simulink library "ammclib_bam_S32K14x"  (R2016a)
settings: Solver=VariableStepAuto  SolverMode=SingleTasking  StartTime=0.0  StopTime=10.0  RelTol=1e-3
undefined symbols (not defined in the file or in its folder): f16A1, f16A2, f16ADCMaxError, f16B0, f16B1, f16B2, f16C1, f16CC1, f16CC1sc, f16CC1sc_D, f16CC1sc_Q, f16CC2, f16CC2sc, f16CC2sc_D, f16CC2sc_Q, f16DerivGain, f16EGain, f16FiltCoef, f16HystOff, f16HystOn, f16IGain, f16IntegGain, f16IntegGainFW, f16IntegGainQ, f16Kd, f16Kq, f16Limit, f16LowerLimit, f16LowerLimit_D, f16LowerLimit_Q, f16LowerLimitFW, f16LowerLimitQ, f16ModIndex, f16OutValOff, f16OutValOn, f16PropGain, f16PropGainFW, f16PropGainQ, f16RampDown, f16RampUp, f16UGain, f16UpperLimit, f16UpperLimit_D, f16UpperLimit_Q, f16UpperLimitFW, f16UpperLimitQ, f16WIGain, f32A1, f32A2, f32ADCMaxError, f32B0, f32B1, f32B2, f32C1, f32CC1, f32CC1sc, f32CC1sc_D, f32CC1sc_Q, f32CC2, f32CC2sc ... (+114)
(part 14 of 22)

== system ammclib_bam_S32K14x/GMCLIB/F16 ==
  GMCLIB_BetaProjection3Ph_F16 : Subsystem  TreatAsAtomicUnit=on  mask(GMCLIB_BetaProjection3Ph_F16){}
      mask help: 3-phase Beta-projection transformation in 16-bit fixed-point fractional implementation. Refer to the AMMCLIB User's Guide for further details.
      mask init: same as ammclib_bam_S32K14x/GDFLIB/F16/GDFLIB_FilterFIR_F16
      settings: RTWSystemCode=Inline
      mask Help: web([fileparts(which('ammclib_bam_S32K14x.slx')) '/../doc/S32K14XMCLUG.pdf'], '-browser')
      mask Display: pos = get_param(gcb, 'Position');width = pos(3) - pos(1); height = pos(4) - pos(2);tX=width/2;tY=height - 8;color('black');text(tX,tY, 'GMCLIB_BetaProjection3Ph_F16', 'horizontalAlignment', 'center');
  GMCLIB_BetaProjection_F16 : Subsystem  TreatAsAtomicUnit=on  mask(GMCLIB_BetaProjection_F16){}
      mask help: Beta Projection transformation 3ph -> 2ph in 16-bit fixed-point fractional implementation. Refer to the AMMCLIB User's Guide for further details.
      mask init: same as ammclib_bam_S32K14x/GDFLIB/F16/GDFLIB_FilterFIR_F16
      settings: RTWSystemCode=Inline
      mask Help: web([fileparts(which('ammclib_bam_S32K14x.slx')) '/../doc/S32K14XMCLUG.pdf'], '-browser')
      mask Display: pos = get_param(gcb, 'Position');width = pos(3) - pos(1); height = pos(4) - pos(2);tX=width/2;tY=height - 8;color('black');text(tX,tY, 'GMCLIB_BetaProjection_F16', 'horizontalAlignment', 'center');
  GMCLIB_ClarkInv_F16 : Subsystem  TreatAsAtomicUnit=on  mask(GMCLIB_ClarkInv_F16){}
      mask help: Inverse Clarke transformation 2ph -> 3ph in 16-bit fixed-point fractional implementation. Refer to the AMMCLIB User's Guide for further details.
      mask init: same as ammclib_bam_S32K14x/GDFLIB/F16/GDFLIB_FilterFIR_F16
      settings: RTWSystemCode=Inline
      mask Help: web([fileparts(which('ammclib_bam_S32K14x.slx')) '/../doc/S32K14XMCLUG.pdf'], '-browser')
      mask Display: pos = get_param(gcb, 'Position');width = pos(3) - pos(1); height = pos(4) - pos(2);tX=width/2;tY=height - 8;color('black');text(tX,tY, 'GMCLIB_ClarkInv_F16', 'horizontalAlignment', 'center');
  GMCLIB_Clark_F16 : Subsystem  TreatAsAtomicUnit=on  mask(GMCLIB_Clark_F16){}
      mask help: Clarke transformation 3ph -> 2ph in 16-bit fixed-point fractional implementation. Refer to the AMMCLIB User's Guide for further details.
      mask init: same as ammclib_bam_S32K14x/GDFLIB/F16/GDFLIB_FilterFIR_F16
      settings: RTWSystemCode=Inline
      mask Help: web([fileparts(which('ammclib_bam_S32K14x.slx')) '/../doc/S32K14XMCLUG.pdf'], '-browser')
      mask Display: pos = get_param(gcb, 'Position');width = pos(3) - pos(1); height = pos(4) - pos(2);tX=width/2;tY=height - 8;color('black');text(tX,tY, 'GMCLIB_Clark_F16', 'horizontalAlignment', 'center');
  GMCLIB_DecouplingPMSM_F16 : Subsystem  TreatAsAtomicUnit=on  mask(GMCLIB_DecouplingPMSM_F16){showStates=Hide (faster execution), f16Kd=0, s16KdShift=0, f16Kq=0, s16KqShift=0}
      mask prompts: showStates "Show internal states"; f16Kd "f16Kd (Coefficient k_d)"; s16KdShift "s16KdShift (Scaling coefficient k_d_shift)"; f16Kq "f16Kq (Coefficient k_q)"; s16KqShift "s16KqShift (Scaling coefficient k_q_shift)"
      mask help: Decoupling of d and q axis of PMSM model in 16-bit fixed-point fractional implementation. Refer to the AMMCLIB User's Guide for further details.
      mask init:
      | if ~evalin('base','exist(''tS8'',''var'')')
      |   if (2 ~= exist('SWLIBS_Typedefs.mat','file'))
      |       error('File SWLIBS_Typedefs.mat is not on the Matlab path. Please add the AMMCLIB "bam" folder in the Matlab Search Path.');
      |   else
      |       evalin('base', 'load(''SWLIBS_Typedefs.mat'')');
      |   end
      | end
      | if showStates == 1
      |     % hidden state variables
      |     if strcmp(get_param([gcb '/f16Kd'], 'BlockType'), 'Inport')
      |         posblk = get_param(gcb, 'Position');
      | 
      |         pos = get_param(    [gcb, '/f16Kd'], 'Position');
      |         orient = get_param( [gcb, '/f16Kd'], 'Orientation');
      |         delete_block(       [gcb, '/f16Kd']);
      |         add_block('built-in/Ground', [gcb, '/f16Kd'], 'Position', pos, 'Orientation', orient);
      | 
      |         pos = get_param(    [gcb, '/s16KdShift'], 'Position');
      |         orient = get_param( [gcb, '/s16KdShift'], 'Orientation');
      |         delete_block(       [gcb, '/s16KdShift']);
      |         add_block('built-in/Ground', [gcb, '/s16KdShift'], 'Position', pos, 'Orientation', orient);
      | 
      |         pos = get_param(    [gcb, '/f16Kq'], 'Position');
      |         orient = get_param( [gcb, '/f16Kq'], 'Orientation');
      |         delete_block(       [gcb, '/f16Kq']);
      |         add_block('built-in/Ground', [gcb, '/f16Kq'], 'Position', pos, 'Orientation', orient);
      | 
      |         pos = get_param(    [gcb, '/s16KqShift'], 'Position');
      |         orient = get_param( [gcb, '/s16KqShift'], 'Orientation');
      |         delete_block(       [gcb, '/s16KqShift']);
      |         add_block('built-in/Ground', [gcb, '/s16KqShift'], 'Position', pos, 'Orientation', orient);
      | 
      | 
      | 
      |         set_param([gcb '/pUdq'], 'Port', '1');
      |         set_param([gcb '/pIdq'], 'Port', '2');
      |         set_param([gcb '/f16AngularVel'], 'Port', '3');
      | 
      |         set_param([gcb '/pUdqDec'], 'Port', '1');
      | 
      |         set_param(gcb,'MaskEnables',{'on','on','on','on','on'});
      | 
      |         if (posblk(4) - posblk(2)) > 100
      |           height = 100;
      |           set_param(gcb,'Position',[posblk(1), posblk(2), posblk(3), posblk(2)+height])
      |         end
      |     end
      | else
      |     % shown state variables
      |     if strcmp(get_param([gcb '/f16Kd'], 'BlockType'), 'Ground')
      |         posblk = get_param(gcb, 'Position');
      | 
      |         pos = get_param(    [gcb, '/f16Kd'], 'Position');
      |         orient = get_param( [gcb, '/f16Kd'], 'Orientation');
      |         delete_block(       [gcb, '/f16Kd']);
      |         add_block('built-in/Inport', [gcb, '/f16Kd'], 'Position', pos, 'Orientation', orient, 'OutDataTypeStr', 'int16');
      | 
      |         pos = get_param(    [gcb, '/s16KdShift'], 'Position');
      |         orient = get_param( [gcb, '/s16KdShift'], 'Orientation');
      |         delete_block(       [gcb, '/s16KdShift']);
      |         add_block('built-in/Inport', [gcb, '/s16KdShift'], 'Position', pos, 'Orientation', orient, 'OutDataTypeStr', 'int16');
      | 
      |         pos = get_param(    [gcb, '/f16Kq'], 'Position');
      |         orient = get_param( [gcb, '/f16Kq'], 'Orientation');
      |         delete_block(       [gcb, '/f16Kq']);
      |         add_block('built-in/Inport', [gcb, '/f16Kq'], 'Position', pos, 'Orientation', orient, 'OutDataTypeStr', 'int16');
      | 
      |         pos = get_param(    [gcb, '/s16KqShift'], 'Position');
      |         orient = get_param( [gcb, '/s16KqShift'], 'Orientation');
      |         delete_block(       [gcb, '/s16KqShift']);
      |         add_block('built-in/Inport', [gcb, '/s16KqShift'], 'Position', pos, 'Orientation', orient, 'OutDataTypeStr', 'int16');
      | 
      | 
      | 
      |         set_param([gcb '/pUdq'], 'Port', '1');
      |         set_param([gcb '/pIdq'], 'Port', '2');
      |         set_param([gcb '/f16AngularVel'], 'Port', '3');
      |         set_param([gcb '/f16Kd'], 'Port', '4');
      |         set_param([gcb '/s16KdShift'], 'Port', '5');
      |         set_param([gcb '/f16Kq'], 'Port', '6');
      |         set_param([gcb '/s16KqShift'], 'Port', '7');
      | 
      |         set_param([gcb '/pUdqDec'], 'Port', '1');
      | 
      |         set_param(gcb,'MaskEnables',{'on','off','off','off','off'});
      | 
      |         if (posblk(4) - posblk(2)) < 200
      |           height = 200;
      |           set_param(gcb,'Position',[posblk(1), posblk(2), posblk(3), posblk(2)+height])
      |         end
      |     end
      | end
      settings: RTWSystemCode=Inline
      mask Help: web([fileparts(which('ammclib_bam_S32K14x.slx')) '/../doc/S32K14XMCLUG.pdf'], '-browser')
      mask TypeOptions showStates: Hide (faster execution) | Show (allows debugging; connect feedback loops manually)
      mask Callback showStates:
      | maskStr = get_param(gcb,'showStates');
      | if strcmp(maskStr,'Hide (faster execution)'),
      |     set_param(gcb,'MaskEnables',{'on','on','on','on','on'});
      | else
      |     set_param(gcb,'MaskEnables',{'on','off','off','off','off'});
      | end
      mask Display:
      | color('black');
      | pos = get_param(gcb, 'Position');
      | width = pos(3) - pos(1);
      | height = pos(4) - pos(2);
      | tX=width/2;
      | tY=height - 8;
      | color('black');
      | text(tX,tY, 'GMCLIB_DecouplingPMSM_F16', 'horizontalAlignment', 'center');
      | if showStates == 2
      |   color('red');
      |   text(tX,tY - 20, ['debugging mode' char(13) char(10) '(limited performance)'], 'horizontalAlignment', 'center');
      | end
  GMCLIB_ElimDcBusRip_F16 : Subsystem  TreatAsAtomicUnit=on  mask(GMCLIB_ElimDcBusRip_F16){showStates=Hide (faster execution), f16ModIndex=0}
      mask prompts: showStates "Show internal states"; f16ModIndex "f16ModIndex (Inverse Modulation Index)"
      mask help: DC Bus voltage ripple elimination function in 16-bit fixed-point fractional implementation. Refer to the AMMCLIB User's Guide for further details.
      mask init:
      | if ~evalin('base','exist(''tS8'',''var'')')
      |   if (2 ~= exist('SWLIBS_Typedefs.mat','file'))
      |       error('File SWLIBS_Typedefs.mat is not on the Matlab path. Please add the AMMCLIB "bam" folder in the Matlab Search Path.');
      |   else
      |       evalin('base', 'load(''SWLIBS_Typedefs.mat'')');
      |   end
      | end
      | if showStates == 1
      |     % hidden state variables
      |     if strcmp(get_param([gcb '/f16ModIndex'], 'BlockType'), 'Inport')
      |         posblk = get_param(gcb, 'Position');
      | 
      |         pos = get_param(    [gcb, '/f16ModIndex'], 'Position');
      |         orient = get_param( [gcb, '/f16ModIndex'], 'Orientation');
      |         delete_block(       [gcb, '/f16ModIndex']);
      |         add_block('built-in/Ground', [gcb, '/f16ModIndex'], 'Position', pos, 'Orientation', orient);
      | 
      | 
      | 
      |         set_param([gcb '/pIn'], 'Port', '1');
      |         set_param([gcb '/f16ArgDcBusMsr'], 'Port', '2');
      | 
      |         set_param([gcb '/pOut'], 'Port', '1');
      | 
      |         set_param(gcb,'MaskEnables',{'on','on'});
      | 
      |         if (posblk(4) - posblk(2)) > 75
      |           height = 75;
      |           set_param(gcb,'Position',[posblk(1), posblk(2), posblk(3), posblk(2)+height])
      |         end
      |     end
      | else
      |     % shown state variables
      |     if strcmp(get_param([gcb '/f16ModIndex'], 'BlockType'), 'Ground')
      |         posblk = get_param(gcb, 'Position');
      | 
      |         pos = get_param(    [gcb, '/f16ModIndex'], 'Position');
      |         orient = get_param( [gcb, '/f16ModIndex'], 'Orientation');
      |         delete_block(       [gcb, '/f16ModIndex']);
      |         add_block('built-in/Inport', [gcb, '/f16ModIndex'], 'Position', pos, 'Orientation', orient, 'OutDataTypeStr', 'int16');
      | 
      | 
      | 
      |         set_param([gcb '/pIn'], 'Port', '1');
      |         set_param([gcb '/f16ArgDcBusMsr'], 'Port', '2');
      |         set_param([gcb '/f16ModIndex'], 'Port', '3');
      | 
      |         set_param([gcb '/pOut'], 'Port', '1');
      | 
      |         set_param(gcb,'MaskEnables',{'on','off'});
      | 
      |         if (posblk(4) - posblk(2)) < 100
      |           height = 100;
      |           set_param(gcb,'Position',[posblk(1), posblk(2), posblk(3), posblk(2)+height])
      |         end
      |     end
      | end
      settings: RTWSystemCode=Inline
      mask Help: web([fileparts(which('ammclib_bam_S32K14x.slx')) '/../doc/S32K14XMCLUG.pdf'], '-browser')
      mask TypeOptions showStates: Hide (faster execution) | Show (allows debugging; connect feedback loops manually)
      mask Callback showStates:
      | maskStr = get_param(gcb,'showStates');
      | if strcmp(maskStr,'Hide (faster execution)'),
      |     set_param(gcb,'MaskEnables',{'on','on'});
      | else
      |     set_param(gcb,'MaskEnables',{'on','off'});
      | end
      mask Display:
      | color('black');
      | pos = get_param(gcb, 'Position');
      | width = pos(3) - pos(1);
      | height = pos(4) - pos(2);
      | tX=width/2;
      | tY=height - 8;
      | color('black');
      | text(tX,tY, 'GMCLIB_ElimDcBusRip_F16', 'horizontalAlignment', 'center');
      | if showStates == 2
      |   color('red');
      |   text(tX,tY - 20, ['debugging mode' char(13) char(10) '(limited performance)'], 'horizontalAlignment', 'center');
      | end
  GMCLIB_ParkInv_F16 : Subsystem  TreatAsAtomicUnit=on  mask(GMCLIB_ParkInv_F16){}
      mask help: Inverse Park transformation 2ph rotational -> 2ph stationary in 16-bit fixed-point fractional implementation. Refer to the AMMCLIB User's Guide for further details.
      mask init: same as ammclib_bam_S32K14x/GDFLIB/F16/GDFLIB_FilterFIR_F16
      settings: RTWSystemCode=Inline
      mask Help: web([fileparts(which('ammclib_bam_S32K14x.slx')) '/../doc/S32K14XMCLUG.pdf'], '-browser')
      mask Display: pos = get_param(gcb, 'Position');width = pos(3) - pos(1); height = pos(4) - pos(2);tX=width/2;tY=height - 8;color('black');text(tX,tY, 'GMCLIB_ParkInv_F16', 'horizontalAlignment', 'center');
  GMCLIB_Park_F16 : Subsystem  TreatAsAtomicUnit=on  mask(GMCLIB_Park_F16){}
      mask help: Park transformation 2ph stationary -> 2ph rotational in 16-bit fixed-point fractional implementation. Refer to the AMMCLIB User's Guide for further details.
      mask init: same as ammclib_bam_S32K14x/GDFLIB/F16/GDFLIB_FilterFIR_F16
      settings: RTWSystemCode=Inline
      mask Help: web([fileparts(which('ammclib_bam_S32K14x.slx')) '/../doc/S32K14XMCLUG.pdf'], '-browser')
      mask Display: pos = get_param(gcb, 'Position');width = pos(3) - pos(1); height = pos(4) - pos(2);tX=width/2;tY=height - 8;color('black');text(tX,tY, 'GMCLIB_Park_F16', 'horizontalAlignment', 'center');
  GMCLIB_PwmIct_F16 : Subsystem  TreatAsAtomicUnit=on  mask(GMCLIB_PwmIct_F16){}
      mask help: General Sinusoidal PWM in 16-bit fixed-point fractional implementation. Refer to the AMMCLIB User's Guide for further details.
      mask init: same as ammclib_bam_S32K14x/GDFLIB/F16/GDFLIB_FilterFIR_F16
      settings: RTWSystemCode=Inline
      mask Help: web([fileparts(which('ammclib_bam_S32K14x.slx')) '/../doc/S32K14XMCLUG.pdf'], '-browser')
      mask Display: pos = get_param(gcb, 'Position');width = pos(3) - pos(1); height = pos(4) - pos(2);tX=width/2;tY=height - 8;color('black');text(tX,tY, 'GMCLIB_PwmIct_F16', 'horizontalAlignment', 'center');
  GMCLIB_SvmSci_F16 : Subsystem  TreatAsAtomicUnit=on  mask(GMCLIB_SvmSci_F16){}
      mask help: General Sinusoidal Modulation with Injection of Third Harmonic in 16-bit fixed-point fractional implementation. Refer to the AMMCLIB User's Guide for further details.
      mask init: same as ammclib_bam_S32K14x/GDFLIB/F16/GDFLIB_FilterFIR_F16
      settings: RTWSystemCode=Inline
      mask Help: web([fileparts(which('ammclib_bam_S32K14x.slx')) '/../doc/S32K14XMCLUG.pdf'], '-browser')
      mask Display: pos = get_param(gcb, 'Position');width = pos(3) - pos(1); height = pos(4) - pos(2);tX=width/2;tY=height - 8;color('black');text(tX,tY, 'GMCLIB_SvmSci_F16', 'horizontalAlignment', 'center');
  GMCLIB_SvmStd_F16 : Subsystem  TreatAsAtomicUnit=on  mask(GMCLIB_SvmStd_F16){}
      mask help: Standard Space Vector Modulation in 16-bit fixed-point fractional implementation. Refer to the AMMCLIB User's Guide for further details.
      mask init: same as ammclib_bam_S32K14x/GDFLIB/F16/GDFLIB_FilterFIR_F16
      settings: RTWSystemCode=Inline
      mask Help: web([fileparts(which('ammclib_bam_S32K14x.slx')) '/../doc/S32K14XMCLUG.pdf'], '-browser')
      mask Display: pos = get_param(gcb, 'Position');width = pos(3) - pos(1); height = pos(4) - pos(2);tX=width/2;tY=height - 8;color('black');text(tX,tY, 'GMCLIB_SvmStd_F16', 'horizontalAlignment', 'center');
  GMCLIB_SvmU0n_F16 : Subsystem  TreatAsAtomicUnit=on  mask(GMCLIB_SvmU0n_F16){}
      mask help: Special Space Vector Modulation with O_000 Nulls in 16-bit fixed-point fractional implementation. Refer to the AMMCLIB User's Guide for further details.
      mask init: same as ammclib_bam_S32K14x/GDFLIB/F16/GDFLIB_FilterFIR_F16
      settings: RTWSystemCode=Inline
      mask Help: web([fileparts(which('ammclib_bam_S32K14x.slx')) '/../doc/S32K14XMCLUG.pdf'], '-browser')
      mask Display: pos = get_param(gcb, 'Position');width = pos(3) - pos(1); height = pos(4) - pos(2);tX=width/2;tY=height - 8;color('black');text(tX,tY, 'GMCLIB_SvmU0n_F16', 'horizontalAlignment', 'center');
  GMCLIB_SvmU7n_F16 : Subsystem  TreatAsAtomicUnit=on  mask(GMCLIB_SvmU7n_F16){}
      mask help: Special Space Vector Modulation with O_111 Ones in 16-bit fixed-point fractional implementation. Refer to the AMMCLIB User's Guide for further details.
      mask init: same as ammclib_bam_S32K14x/GDFLIB/F16/GDFLIB_FilterFIR_F16
      settings: RTWSystemCode=Inline
      mask Help: web([fileparts(which('ammclib_bam_S32K14x.slx')) '/../doc/S32K14XMCLUG.pdf'], '-browser')
      mask Display: pos = get_param(gcb, 'Position');width = pos(3) - pos(1); height = pos(4) - pos(2);tX=width/2;tY=height - 8;color('black');text(tX,tY, 'GMCLIB_SvmU7n_F16', 'horizontalAlignment', 'center');
  GMCLIB_VRot_F16 : Subsystem  TreatAsAtomicUnit=on  mask(GMCLIB_VRot_F16){}
      mask help: Vector rotation in 16-bit fixed-point fractional implementation.
      mask init: same as ammclib_bam_S32K14x/GDFLIB/F16/GDFLIB_FilterFIR_F16
      settings: RTWSystemCode=Inline
      mask Help: web([fileparts(which('ammclib_bam_S32K14x.slx')) '/../doc/S32K14XMCLUG.pdf'], '-browser')
      mask Display: pos = get_param(gcb, 'Position');width = pos(3) - pos(1); height = pos(4) - pos(2);tX=width/2;tY=height - 8;color('black');text(tX,tY, 'GMCLIB_VRot_F16', 'horizontalAlignment', 'center');
  GMCLIB_VUnit_F16 : Subsystem  TreatAsAtomicUnit=on  mask(GMCLIB_VUnit_F16){}
      mask help: Vector normalization in 16-bit fixed-point fractional implementation.
      mask init: same as ammclib_bam_S32K14x/GDFLIB/F16/GDFLIB_FilterFIR_F16
      settings: RTWSystemCode=Inline
      mask Help: web([fileparts(which('ammclib_bam_S32K14x.slx')) '/../doc/S32K14XMCLUG.pdf'], '-browser')
      mask Display: pos = get_param(gcb, 'Position');width = pos(3) - pos(1); height = pos(4) - pos(2);tX=width/2;tY=height - 8;color('black');text(tX,tY, 'GMCLIB_VUnit_F16', 'horizontalAlignment', 'center');
  GMCLIB_Vpol2xy_F16 : Subsystem  TreatAsAtomicUnit=on  mask(GMCLIB_Vpol2xy_F16){}
      mask help: Transformation of polar coordinate system to Cartesian in 16-bit fixed-point fractional implementation.
      mask init: same as ammclib_bam_S32K14x/GDFLIB/F16/GDFLIB_FilterFIR_F16
      settings: RTWSystemCode=Inline
      mask Help: web([fileparts(which('ammclib_bam_S32K14x.slx')) '/../doc/S32K14XMCLUG.pdf'], '-browser')
      mask Display: pos = get_param(gcb, 'Position');width = pos(3) - pos(1); height = pos(4) - pos(2);tX=width/2;tY=height - 8;color('black');text(tX,tY, 'GMCLIB_Vpol2xy_F16', 'horizontalAlignment', 'center');
  GMCLIB_Vxy2pol_F16 : Subsystem  TreatAsAtomicUnit=on  mask(GMCLIB_Vxy2pol_F16){}
      mask help: Transformation of Cartesian coordinate system to polar in 16-bit fixed-point fractional implementation.
      mask init: same as ammclib_bam_S32K14x/GDFLIB/F16/GDFLIB_FilterFIR_F16
      settings: RTWSystemCode=Inline
      mask Help: web([fileparts(which('ammclib_bam_S32K14x.slx')) '/../doc/S32K14XMCLUG.pdf'], '-browser')
      mask Display: pos = get_param(gcb, 'Position');width = pos(3) - pos(1); height = pos(4) - pos(2);tX=width/2;tY=height - 8;color('black');text(tX,tY, 'GMCLIB_Vxy2pol_F16', 'horizontalAlignment', 'center');

== system ammclib_bam_S32K14x/GMCLIB/F32 ==
  GMCLIB_BetaProjection3Ph_F32 : Subsystem  TreatAsAtomicUnit=on  mask(GMCLIB_BetaProjection3Ph_F32){}
      mask help: 3-phase Beta-projection transformation in 32-bit fixed-point fractional implementation. Refer to the AMMCLIB User's Guide for further details.
      mask init: same as ammclib_bam_S32K14x/GDFLIB/F16/GDFLIB_FilterFIR_F16
      settings: RTWSystemCode=Inline
      mask Help: web([fileparts(which('ammclib_bam_S32K14x.slx')) '/../doc/S32K14XMCLUG.pdf'], '-browser')
      mask Display: pos = get_param(gcb, 'Position');width = pos(3) - pos(1); height = pos(4) - pos(2);tX=width/2;tY=height - 8;color('black');text(tX,tY, 'GMCLIB_BetaProjection3Ph_F32', 'horizontalAlignment', 'center');
  GMCLIB_BetaProjection_F32 : Subsystem  TreatAsAtomicUnit=on  mask(GMCLIB_BetaProjection_F32){}
      mask help: Beta Projection transformation 3ph -> 2ph in 32-bit fixed-point fractional implementation. Refer to the AMMCLIB User's Guide for further details.
      mask init: same as ammclib_bam_S32K14x/GDFLIB/F16/GDFLIB_FilterFIR_F16
      settings: RTWSystemCode=Inline
      mask Help: web([fileparts(which('ammclib_bam_S32K14x.slx')) '/../doc/S32K14XMCLUG.pdf'], '-browser')
      mask Display: pos = get_param(gcb, 'Position');width = pos(3) - pos(1); height = pos(4) - pos(2);tX=width/2;tY=height - 8;color('black');text(tX,tY, 'GMCLIB_BetaProjection_F32', 'horizontalAlignment', 'center');
  GMCLIB_ClarkInv_F32 : Subsystem  TreatAsAtomicUnit=on  mask(GMCLIB_ClarkInv_F32){}
      mask help: Inverse Clarke transformation 2ph -> 3ph in 32-bit fixed-point fractional implementation. Refer to the AMMCLIB User's Guide for further details.
      mask init: same as ammclib_bam_S32K14x/GDFLIB/F16/GDFLIB_FilterFIR_F16
      settings: RTWSystemCode=Inline
      mask Help: web([fileparts(which('ammclib_bam_S32K14x.slx')) '/../doc/S32K14XMCLUG.pdf'], '-browser')
      mask Display: pos = get_param(gcb, 'Position');width = pos(3) - pos(1); height = pos(4) - pos(2);tX=width/2;tY=height - 8;color('black');text(tX,tY, 'GMCLIB_ClarkInv_F32', 'horizontalAlignment', 'center');
  GMCLIB_Clark_F32 : Subsystem  TreatAsAtomicUnit=on  mask(GMCLIB_Clark_F32){}
      mask help: Clarke transformation 3ph -> 2ph in 32-bit fixed-point fractional implementation. Refer to the AMMCLIB User's Guide for further details.
      mask init: same as ammclib_bam_S32K14x/GDFLIB/F16/GDFLIB_FilterFIR_F16
      settings: RTWSystemCode=Inline
      mask Help: web([fileparts(which('ammclib_bam_S32K14x.slx')) '/../doc/S32K14XMCLUG.pdf'], '-browser')
      mask Display: pos = get_param(gcb, 'Position');width = pos(3) - pos(1); height = pos(4) - pos(2);tX=width/2;tY=height - 8;color('black');text(tX,tY, 'GMCLIB_Clark_F32', 'horizontalAlignment', 'center');
  GMCLIB_DecouplingPMSM_F32 : Subsystem  TreatAsAtomicUnit=on  mask(GMCLIB_DecouplingPMSM_F32){showStates=Hide (faster execution), f32Kd=0, s16KdShift=0, f32Kq=0, s16KqShift=0}
      mask prompts: showStates "Show internal states"; f32Kd "f32Kd (Coefficient k_d)"; s16KdShift "s16KdShift (Scaling coefficient k_d_shift)"; f32Kq "f32Kq (Coefficient k_q)"; s16KqShift "s16KqShift (Scaling coefficient k_q_shift)"
      mask help: Decoupling of d and q axis of PMSM model in 32-bit fixed-point fractional implementation. Refer to the AMMCLIB User's Guide for further details.
      mask init:
      | if ~evalin('base','exist(''tS8'',''var'')')
      |   if (2 ~= exist('SWLIBS_Typedefs.mat','file'))
      |       error('File SWLIBS_Typedefs.mat is not on the Matlab path. Please add the AMMCLIB "bam" folder in the Matlab Search Path.');
      |   else
      |       evalin('base', 'load(''SWLIBS_Typedefs.mat'')');
      |   end
      | end
      | if showStates == 1
      |     % hidden state variables
      |     if strcmp(get_param([gcb '/f32Kd'], 'BlockType'), 'Inport')
      |         posblk = get_param(gcb, 'Position');
      | 
      |         pos = get_param(    [gcb, '/f32Kd'], 'Position');
      |         orient = get_param( [gcb, '/f32Kd'], 'Orientation');
      |         delete_block(       [gcb, '/f32Kd']);
      |         add_block('built-in/Ground', [gcb, '/f32Kd'], 'Position', pos, 'Orientation', orient);
      | 
      |         pos = get_param(    [gcb, '/s16KdShift'], 'Position');
      |         orient = get_param( [gcb, '/s16KdShift'], 'Orientation');
      |         delete_block(       [gcb, '/s16KdShift']);
      |         add_block('built-in/Ground', [gcb, '/s16KdShift'], 'Position', pos, 'Orientation', orient);
      | 
      |         pos = get_param(    [gcb, '/f32Kq'], 'Position');
      |         orient = get_param( [gcb, '/f32Kq'], 'Orientation');
      |         delete_block(       [gcb, '/f32Kq']);
      |         add_block('built-in/Ground', [gcb, '/f32Kq'], 'Position', pos, 'Orientation', orient);
      | 
      |         pos = get_param(    [gcb, '/s16KqShift'], 'Position');
      |         orient = get_param( [gcb, '/s16KqShift'], 'Orientation');
      |         delete_block(       [gcb, '/s16KqShift']);
      |         add_block('built-in/Ground', [gcb, '/s16KqShift'], 'Position', pos, 'Orientation', orient);
      | 
      | 
      | 
      |         set_param([gcb '/pUdq'], 'Port', '1');
      |         set_param([gcb '/pIdq'], 'Port', '2');
      |         set_param([gcb '/f32AngularVel'], 'Port', '3');
      | 
      |         set_param([gcb '/pUdqDec'], 'Port', '1');
      | 
      |         set_param(gcb,'MaskEnables',{'on','on','on','on','on'});
      | 
      |         if (posblk(4) - posblk(2)) > 100
      |           height = 100;
      |           set_param(gcb,'Position',[posblk(1), posblk(2), posblk(3), posblk(2)+height])
      |         end
      |     end
      | else
      |     % shown state variables
      |     if strcmp(get_param([gcb '/f32Kd'], 'BlockType'), 'Ground')
      |         posblk = get_param(gcb, 'Position');
      | 
      |         pos = get_param(    [gcb, '/f32Kd'], 'Position');
      |         orient = get_param( [gcb, '/f32Kd'], 'Orientation');
      |         delete_block(       [gcb, '/f32Kd']);
      |         add_block('built-in/Inport', [gcb, '/f32Kd'], 'Position', pos, 'Orientation', orient, 'OutDataTypeStr', 'int32');
      | 
      |         pos = get_param(    [gcb, '/s16KdShift'], 'Position');
      |         orient = get_param( [gcb, '/s16KdShift'], 'Orientation');
      |         delete_block(       [gcb, '/s16KdShift']);
      |         add_block('built-in/Inport', [gcb, '/s16KdShift'], 'Position', pos, 'Orientation', orient, 'OutDataTypeStr', 'int16');
      | 
      |         pos = get_param(    [gcb, '/f32Kq'], 'Position');
      |         orient = get_param( [gcb, '/f32Kq'], 'Orientation');
      |         delete_block(       [gcb, '/f32Kq']);
      |         add_block('built-in/Inport', [gcb, '/f32Kq'], 'Position', pos, 'Orientation', orient, 'OutDataTypeStr', 'int32');
      | 
      |         pos = get_param(    [gcb, '/s16KqShift'], 'Position');
      |         orient = get_param( [gcb, '/s16KqShift'], 'Orientation');
      |         delete_block(       [gcb, '/s16KqShift']);
      |         add_block('built-in/Inport', [gcb, '/s16KqShift'], 'Position', pos, 'Orientation', orient, 'OutDataTypeStr', 'int16');
      | 
      | 
      | 
      |         set_param([gcb '/pUdq'], 'Port', '1');
      |         set_param([gcb '/pIdq'], 'Port', '2');
      |         set_param([gcb '/f32AngularVel'], 'Port', '3');
      |         set_param([gcb '/f32Kd'], 'Port', '4');
      |         set_param([gcb '/s16KdShift'], 'Port', '5');
      |         set_param([gcb '/f32Kq'], 'Port', '6');
      |         set_param([gcb '/s16KqShift'], 'Port', '7');
      | 
      |         set_param([gcb '/pUdqDec'], 'Port', '1');
      | 
      |         set_param(gcb,'MaskEnables',{'on','off','off','off','off'});
      | 
      |         if (posblk(4) - posblk(2)) < 200
      |           height = 200;
      |           set_param(gcb,'Position',[posblk(1), posblk(2), posblk(3), posblk(2)+height])
      |         end
      |     end
      | end
      settings: RTWSystemCode=Inline
      mask Help: web([fileparts(which('ammclib_bam_S32K14x.slx')) '/../doc/S32K14XMCLUG.pdf'], '-browser')
      mask TypeOptions showStates: Hide (faster execution) | Show (allows debugging; connect feedback loops manually)
      mask Callback showStates:
      | maskStr = get_param(gcb,'showStates');
      | if strcmp(maskStr,'Hide (faster execution)'),
      |     set_param(gcb,'MaskEnables',{'on','on','on','on','on'});
      | else
      |     set_param(gcb,'MaskEnables',{'on','off','off','off','off'});
      | end
      mask Display:
      | color('black');
      | pos = get_param(gcb, 'Position');
      | width = pos(3) - pos(1);
      | height = pos(4) - pos(2);
      | tX=width/2;
      | tY=height - 8;
      | color('black');
      | text(tX,tY, 'GMCLIB_DecouplingPMSM_F32', 'horizontalAlignment', 'center');
      | if showStates == 2
      |   color('red');
      |   text(tX,tY - 20, ['debugging mode' char(13) char(10) '(limited performance)'], 'horizontalAlignment', 'center');
      | end
  GMCLIB_ElimDcBusRip_F32 : Subsystem  TreatAsAtomicUnit=on  mask(GMCLIB_ElimDcBusRip_F32){showStates=Hide (faster execution), f32ModIndex=0}
      mask prompts: showStates "Show internal states"; f32ModIndex "f32ModIndex (Inverse Modulation Index)"
      mask help: DC Bus voltage ripple elimination function in 32-bit fixed-point fractional implementation. Refer to the AMMCLIB User's Guide for further details.
      mask init:
      | if ~evalin('base','exist(''tS8'',''var'')')
      |   if (2 ~= exist('SWLIBS_Typedefs.mat','file'))
      |       error('File SWLIBS_Typedefs.mat is not on the Matlab path. Please add the AMMCLIB "bam" folder in the Matlab Search Path.');
      |   else
      |       evalin('base', 'load(''SWLIBS_Typedefs.mat'')');
      |   end
      | end
      | if showStates == 1
      |     % hidden state variables
      |     if strcmp(get_param([gcb '/f32ModIndex'], 'BlockType'), 'Inport')
      |         posblk = get_param(gcb, 'Position');
      | 
      |         pos = get_param(    [gcb, '/f32ModIndex'], 'Position');
      |         orient = get_param( [gcb, '/f32ModIndex'], 'Orientation');
      |         delete_block(       [gcb, '/f32ModIndex']);
      |         add_block('built-in/Ground', [gcb, '/f32ModIndex'], 'Position', pos, 'Orientation', orient);
      | 
      | 
      | 
      |         set_param([gcb '/pIn'], 'Port', '1');
      |         set_param([gcb '/f32ArgDcBusMsr'], 'Port', '2');
      | 
      |         set_param([gcb '/pOut'], 'Port', '1');
      | 
      |         set_param(gcb,'MaskEnables',{'on','on'});
      | 
      |         if (posblk(4) - posblk(2)) > 75
      |           height = 75;
      |           set_param(gcb,'Position',[posblk(1), posblk(2), posblk(3), posblk(2)+height])
      |         end
      |     end
      | else
      |     % shown state variables
      |     if strcmp(get_param([gcb '/f32ModIndex'], 'BlockType'), 'Ground')
      |         posblk = get_param(gcb, 'Position');
      | 
      |         pos = get_param(    [gcb, '/f32ModIndex'], 'Position');
      |         orient = get_param( [gcb, '/f32ModIndex'], 'Orientation');
      |         delete_block(       [gcb, '/f32ModIndex']);
      |         add_block('built-in/Inport', [gcb, '/f32ModIndex'], 'Position', pos, 'Orientation', orient, 'OutDataTypeStr', 'int32');
      | 
      | 
      | 
      |         set_param([gcb '/pIn'], 'Port', '1');
      |         set_param([gcb '/f32ArgDcBusMsr'], 'Port', '2');
      |         set_param([gcb '/f32ModIndex'], 'Port', '3');
      | 
      |         set_param([gcb '/pOut'], 'Port', '1');
      | 
      |         set_param(gcb,'MaskEnables',{'on','off'});
      | 
      |         if (posblk(4) - posblk(2)) < 100
      |           height = 100;
      |           set_param(gcb,'Position',[posblk(1), posblk(2), posblk(3), posblk(2)+height])
      |         end
      |     end
      | end
      settings: RTWSystemCode=Inline
      mask Help: web([fileparts(which('ammclib_bam_S32K14x.slx')) '/../doc/S32K14XMCLUG.pdf'], '-browser')
      mask TypeOptions showStates: Hide (faster execution) | Show (allows debugging; connect feedback loops manually)
      mask Callback showStates:
      | maskStr = get_param(gcb,'showStates');
      | if strcmp(maskStr,'Hide (faster execution)'),
      |     set_param(gcb,'MaskEnables',{'on','on'});
      | else
      |     set_param(gcb,'MaskEnables',{'on','off'});
      | end
      mask Display:
      | color('black');
      | pos = get_param(gcb, 'Position');
      | width = pos(3) - pos(1);
      | height = pos(4) - pos(2);
      | tX=width/2;
      | tY=height - 8;
      | color('black');
      | text(tX,tY, 'GMCLIB_ElimDcBusRip_F32', 'horizontalAlignment', 'center');
      | if showStates == 2
      |   color('red');
      |   text(tX,tY - 20, ['debugging mode' char(13) char(10) '(limited performance)'], 'horizontalAlignment', 'center');
      | end
  GMCLIB_ParkInv_F32 : Subsystem  TreatAsAtomicUnit=on  mask(GMCLIB_ParkInv_F32){}
      mask help: Inverse Park transformation 2ph rotational -> 2ph stationary in 32-bit fixed-point fractional implementation. Refer to the AMMCLIB User's Guide for further details.
      mask init: same as ammclib_bam_S32K14x/GDFLIB/F16/GDFLIB_FilterFIR_F16
      settings: RTWSystemCode=Inline
      mask Help: web([fileparts(which('ammclib_bam_S32K14x.slx')) '/../doc/S32K14XMCLUG.pdf'], '-browser')
      mask Display: pos = get_param(gcb, 'Position');width = pos(3) - pos(1); height = pos(4) - pos(2);tX=width/2;tY=height - 8;color('black');text(tX,tY, 'GMCLIB_ParkInv_F32', 'horizontalAlignment', 'center');
  GMCLIB_Park_F32 : Subsystem  TreatAsAtomicUnit=on  mask(GMCLIB_Park_F32){}
      mask help: Park transformation 2ph stationary -> 2ph rotational in 32-bit fixed-point fractional implementation. Refer to the AMMCLIB User's Guide for further details.
      mask init: same as ammclib_bam_S32K14x/GDFLIB/F16/GDFLIB_FilterFIR_F16
      settings: RTWSystemCode=Inline
      mask Help: web([fileparts(which('ammclib_bam_S32K14x.slx')) '/../doc/S32K14XMCLUG.pdf'], '-browser')
      mask Display: pos = get_param(gcb, 'Position');width = pos(3) - pos(1); height = pos(4) - pos(2);tX=width/2;tY=height - 8;color('black');text(tX,tY, 'GMCLIB_Park_F32', 'horizontalAlignment', 'center');
  GMCLIB_PwmIct_F32 : Subsystem  TreatAsAtomicUnit=on  mask(GMCLIB_PwmIct_F32){}
      mask help: General Sinusoidal PWM in 32-bit fixed-point fractional implementation. Refer to the AMMCLIB User's Guide for further details.
      mask init: same as ammclib_bam_S32K14x/GDFLIB/F16/GDFLIB_FilterFIR_F16
      settings: RTWSystemCode=Inline
      mask Help: web([fileparts(which('ammclib_bam_S32K14x.slx')) '/../doc/S32K14XMCLUG.pdf'], '-browser')
      mask Display: pos = get_param(gcb, 'Position');width = pos(3) - pos(1); height = pos(4) - pos(2);tX=width/2;tY=height - 8;color('black');text(tX,tY, 'GMCLIB_PwmIct_F32', 'horizontalAlignment', 'center');
  GMCLIB_SvmSci_F32 : Subsystem  TreatAsAtomicUnit=on  mask(GMCLIB_SvmSci_F32){}
      mask help: General Sinusoidal Modulation with Injection of Third Harmonic in 32-bit fixed-point fractional implementation. Refer to the AMMCLIB User's Guide for further details.
      mask init: same as ammclib_bam_S32K14x/GDFLIB/F16/GDFLIB_FilterFIR_F16
      settings: RTWSystemCode=Inline
      mask Help: web([fileparts(which('ammclib_bam_S32K14x.slx')) '/../doc/S32K14XMCLUG.pdf'], '-browser')
      mask Display: pos = get_param(gcb, 'Position');width = pos(3) - pos(1); height = pos(4) - pos(2);tX=width/2;tY=height - 8;color('black');text(tX,tY, 'GMCLIB_SvmSci_F32', 'horizontalAlignment', 'center');
  GMCLIB_SvmStd_F32 : Subsystem  TreatAsAtomicUnit=on  mask(GMCLIB_SvmStd_F32){}
      mask help: Standard Space Vector Modulation in 32-bit fixed-point fractional implementation. Refer to the AMMCLIB User's Guide for further details.
      mask init: same as ammclib_bam_S32K14x/GDFLIB/F16/GDFLIB_FilterFIR_F16
      settings: RTWSystemCode=Inline
      mask Help: web([fileparts(which('ammclib_bam_S32K14x.slx')) '/../doc/S32K14XMCLUG.pdf'], '-browser')
      mask Display: pos = get_param(gcb, 'Position');width = pos(3) - pos(1); height = pos(4) - pos(2);tX=width/2;tY=height - 8;color('black');text(tX,tY, 'GMCLIB_SvmStd_F32', 'horizontalAlignment', 'center');
  GMCLIB_SvmU0n_F32 : Subsystem  TreatAsAtomicUnit=on  mask(GMCLIB_SvmU0n_F32){}
      mask help: Special Space Vector Modulation with O_000 Nulls in 32-bit fixed-point fractional implementation. Refer to the AMMCLIB User's Guide for further details.
      mask init: same as ammclib_bam_S32K14x/GDFLIB/F16/GDFLIB_FilterFIR_F16
      settings: RTWSystemCode=Inline
      mask Help: web([fileparts(which('ammclib_bam_S32K14x.slx')) '/../doc/S32K14XMCLUG.pdf'], '-browser')
      mask Display: pos = get_param(gcb, 'Position');width = pos(3) - pos(1); height = pos(4) - pos(2);tX=width/2;tY=height - 8;color('black');text(tX,tY, 'GMCLIB_SvmU0n_F32', 'horizontalAlignment', 'center');
  GMCLIB_SvmU7n_F32 : Subsystem  TreatAsAtomicUnit=on  mask(GMCLIB_SvmU7n_F32){}
      mask help: Special Space Vector Modulation with O_111 Ones in 32-bit fixed-point fractional implementation. Refer to the AMMCLIB User's Guide for further details.
      mask init: same as ammclib_bam_S32K14x/GDFLIB/F16/GDFLIB_FilterFIR_F16
      settings: RTWSystemCode=Inline
      mask Help: web([fileparts(which('ammclib_bam_S32K14x.slx')) '/../doc/S32K14XMCLUG.pdf'], '-browser')
      mask Display: pos = get_param(gcb, 'Position');width = pos(3) - pos(1); height = pos(4) - pos(2);tX=width/2;tY=height - 8;color('black');text(tX,tY, 'GMCLIB_SvmU7n_F32', 'horizontalAlignment', 'center');
  GMCLIB_VRot_F32 : Subsystem  TreatAsAtomicUnit=on  mask(GMCLIB_VRot_F32){}
      mask help: Vector rotation in 32-bit fixed-point fractional implementation.
      mask init: same as ammclib_bam_S32K14x/GDFLIB/F16/GDFLIB_FilterFIR_F16
      settings: RTWSystemCode=Inline
      mask Help: web([fileparts(which('ammclib_bam_S32K14x.slx')) '/../doc/S32K14XMCLUG.pdf'], '-browser')
      mask Display: pos = get_param(gcb, 'Position');width = pos(3) - pos(1); height = pos(4) - pos(2);tX=width/2;tY=height - 8;color('black');text(tX,tY, 'GMCLIB_VRot_F32', 'horizontalAlignment', 'center');
  GMCLIB_VUnit_F32 : Subsystem  TreatAsAtomicUnit=on  mask(GMCLIB_VUnit_F32){}
      mask help: Vector normalization in 32-bit fixed-point fractional implementation.
      mask init: same as ammclib_bam_S32K14x/GDFLIB/F16/GDFLIB_FilterFIR_F16
      settings: RTWSystemCode=Inline
      mask Help: web([fileparts(which('ammclib_bam_S32K14x.slx')) '/../doc/S32K14XMCLUG.pdf'], '-browser')
      mask Display: pos = get_param(gcb, 'Position');width = pos(3) - pos(1); height = pos(4) - pos(2);tX=width/2;tY=height - 8;color('black');text(tX,tY, 'GMCLIB_VUnit_F32', 'horizontalAlignment', 'center');
  GMCLIB_Vpol2xy_F32 : Subsystem  TreatAsAtomicUnit=on  mask(GMCLIB_Vpol2xy_F32){}
      mask help: Transformation of polar coordinate system to Cartesian in 32-bit fixed-point fractional implementation.
      mask init: same as ammclib_bam_S32K14x/GDFLIB/F16/GDFLIB_FilterFIR_F16
      settings: RTWSystemCode=Inline
      mask Help: web([fileparts(which('ammclib_bam_S32K14x.slx')) '/../doc/S32K14XMCLUG.pdf'], '-browser')
      mask Display: pos = get_param(gcb, 'Position');width = pos(3) - pos(1); height = pos(4) - pos(2);tX=width/2;tY=height - 8;color('black');text(tX,tY, 'GMCLIB_Vpol2xy_F32', 'horizontalAlignment', 'center');
  GMCLIB_Vxy2pol_F32 : Subsystem  TreatAsAtomicUnit=on  mask(GMCLIB_Vxy2pol_F32){}
      mask help: Transformation of Cartesian coordinate system to polar in 32-bit fixed-point fractional implementation.
      mask init: same as ammclib_bam_S32K14x/GDFLIB/F16/GDFLIB_FilterFIR_F16
      settings: RTWSystemCode=Inline
      mask Help: web([fileparts(which('ammclib_bam_S32K14x.slx')) '/../doc/S32K14XMCLUG.pdf'], '-browser')
      mask Display: pos = get_param(gcb, 'Position');width = pos(3) - pos(1); height = pos(4) - pos(2);tX=width/2;tY=height - 8;color('black');text(tX,tY, 'GMCLIB_Vxy2pol_F32', 'horizontalAlignment', 'center');
